simulink model "lab1"  (R2023b)
settings: Solver=ode113  StartTime=0.0  StopTime=10.0  RelTol=1e-10
values from neighbouring files (symbols this model uses):
  g = 9.81    [lab0.m]
  theta1 = 3.1    [lab0.m]
  theta2 = 9.5    [lab0.m]
  theta3 = 0.24    [lab0.m]
  theta4 = 0.77    [lab0.m]
settings Model: Creator=alozins2  LastModifiedBy=alozins2

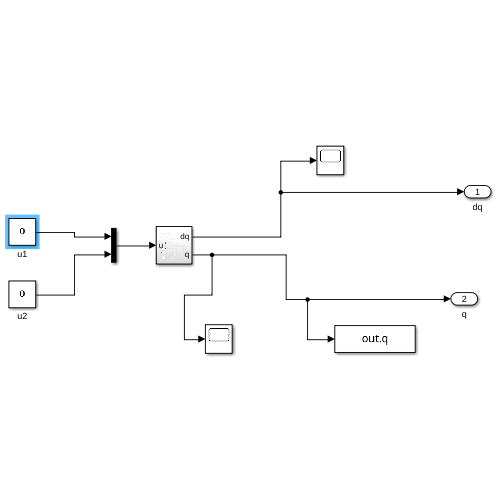
[thumbnail: Simulink's stored preview of the top-level diagram]
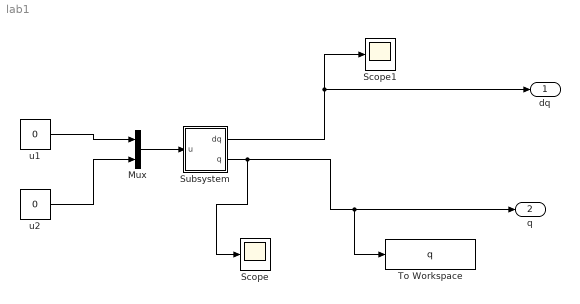
== system lab1 ==
  Mux : Mux  Inputs=2
  Scope : Scope
  Scope1 : Scope
  Subsystem : Subsystem
  To Workspace : ToWorkspace  VariableName=q  SampleTime=-1
  u1 : Constant  Value=0
  u2 : Constant  Value=0
  dq : Outport
  q : Outport  Port=2
  wires:
  Mux/1 -> Subsystem/1(u)
  Subsystem/1(dq) -> Scope1/1, dq/1
  Subsystem/2(q) -> Scope/1, To Workspace/1, q/1
  u1/1 -> Mux/1
  u2/1 -> Mux/2

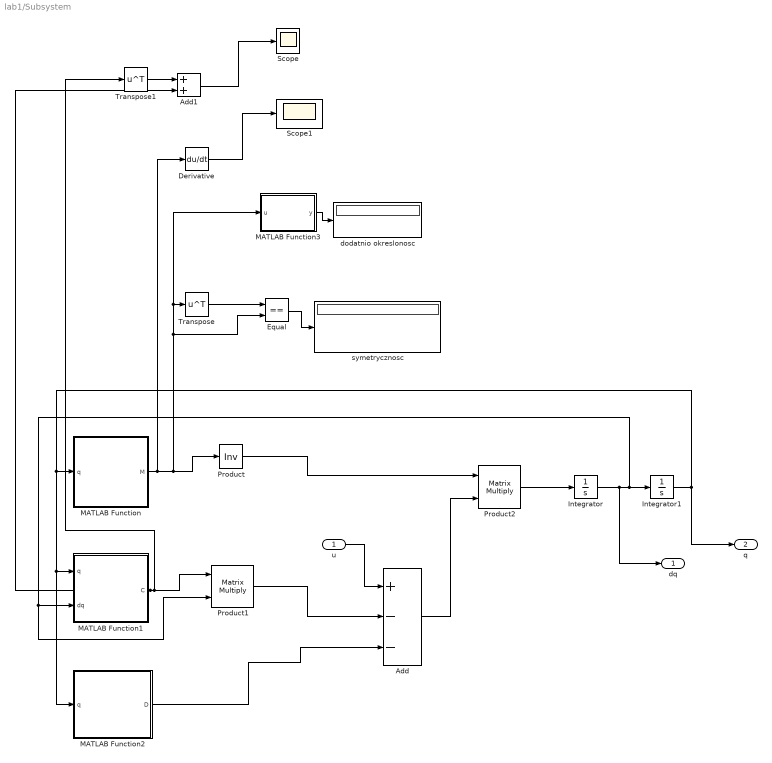
== system lab1/Subsystem ==
  u : Inport
  Add : Sum  Inputs=+--
  Add1 : Sum
  Derivative : Derivative
  Equal : RelationalOperator  Operator===  OutDataTypeStr=boolean  RndMeth=Simplest  InputSameDT=off
  Integrator : Integrator  InitialCondition=[0;0]
  Integrator1 : Integrator  InitialCondition=[-3.14/2;0]
  MATLAB Function : MATLAB Function  TreatAsAtomicUnit=on
  MATLAB Function1 : MATLAB Function  TreatAsAtomicUnit=on
  MATLAB Function2 : MATLAB Function  TreatAsAtomicUnit=on
  MATLAB Function3 : MATLAB Function  TreatAsAtomicUnit=on
  Product : Product  Inputs=/  Multiplication=Matrix(*)
  Product1 : Product  Multiplication=Matrix(*)
  Product2 : Product  Multiplication=Matrix(*)
  Scope : Scope
  Scope1 : Scope
  Transpose : Math  Operator=transpose
  Transpose1 : Math  Operator=transpose
  dodatnio okreslonosc : Display
  symetrycznosc : Display
  dq : Outport
  q : Outport  Port=2
  wires:
  MATLAB Function2/1(D) -> Add/3
  Product1/1 -> Add/2
  MATLAB Function/1(M) -> Derivative/1, Equal/2, MATLAB Function3/1(u), Transpose/1, Product/1
  Product2/1 -> Integrator/1
  MATLAB Function1/1(C) -> Product1/1, Transpose1/1, Add1/2
  Integrator/1 -> dq/1, Product1/2, MATLAB Function1/2(dq), Integrator1/1
  Product/1 -> Product2/1
  u/1 -> Add/1
  Add/1 -> Product2/2
  Integrator1/1 -> q/1, MATLAB Function2/1(q), MATLAB Function1/1(q), MATLAB Function/1(q)
  Transpose/1 -> Equal/1
  Equal/1 -> symetrycznosc/1
  MATLAB Function3/1(y) -> dodatnio okreslonosc/1
  Transpose1/1 -> Add1/1
  Add1/1 -> Scope/1
  Derivative/1 -> Scope1/1

== matlab function lab1/Subsystem/MATLAB Function1 ==
  data: q input; dq input; C output; theta1 parameter; theta3 parameter; theta4 parameter
function C = Corliolis(q,dq,theta1, theta3, theta4)

q1=q(1);
q2=q(2);

dq1=dq(1);
dq2=dq(2);

C=[-dq2, -(dq1+dq2);
    dq1,0]*0.3*theta4*sin(q2);

== matlab function lab1/Subsystem/MATLAB Function ==
  data: q input; M output; theta1 parameter; theta3 parameter; theta4 parameter
function M = interiaMatrix(q,theta1, theta3, theta4)

q1=q(1);
q2=q(2);

M=[theta1 + 0.6*theta4*cos(q2), theta3 + 0.3*theta4*cos(q2);
    theta3 + 0.3*theta4*cos(q2), theta3];

== matlab function lab1/Subsystem/MATLAB Function2 ==
  data: q input; D output; g parameter; theta2 parameter; theta4 parameter
function D = Gravity(q,g,theta2,theta4)

q1=q(1);
q2=q(2);

D=g*[theta2*cos(q1) + theta4*cos(q1+q2);
    theta4*cos(q1+q2)];

== matlab function lab1/Subsystem/MATLAB Function3 ==
  data: u input; y output
function y = fcn(u)

y = det(u);
